simulink model "point_model"  (R2021b)
settings: Solver=VariableStepAuto  StartTime=0.0  StopTime=10.0  RelTol=1e-3
libraries: simulink_extras x4, simulink x2
settings Model: Creator=frederic  LastModifiedBy=frederic

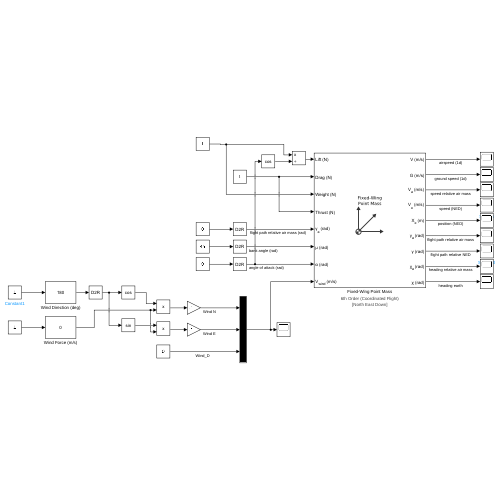
[thumbnail: Simulink's stored preview of the top-level diagram]
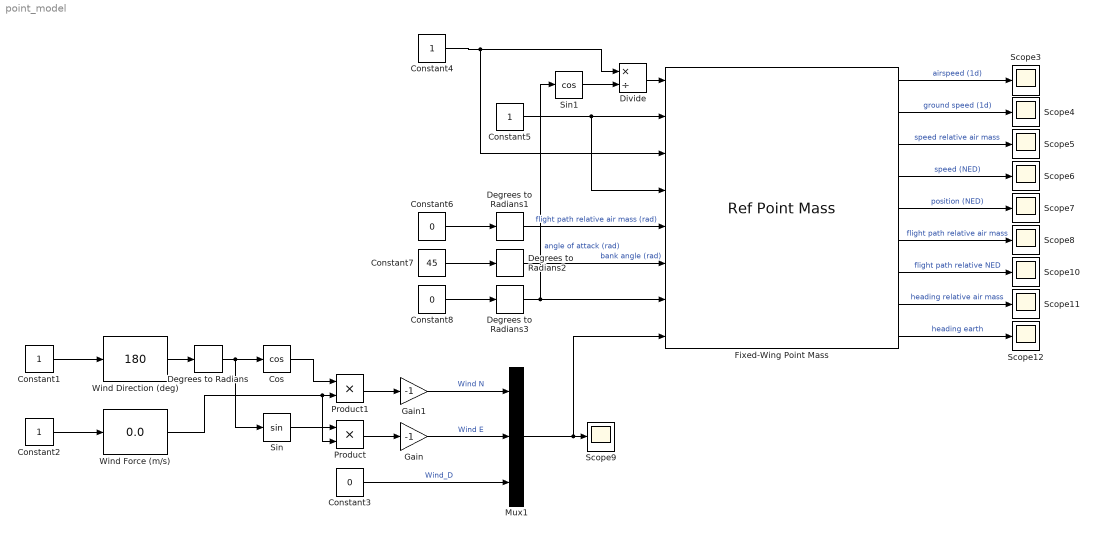
== system point_model ==
  Constant{1..2,4..5} (4 alike) : Constant
  Constant3 : Constant  Value=0
  Constant6 : Constant  Value=0
  Constant7 : Constant  Value=45
  Constant8 : Constant  Value=0
  Cos : Trigonometry  Operator=cos
  Degrees to Radians{,1..3} (4 alike) : simulink_extras/Transformations/Degrees to Radians
  Divide : Product  Inputs=*/
  Fixed-Wing Point Mass : RefPointMass  airspeed=10  mass=1
      settings: AttributesFormatString=|
      | %<order>
      | %<frame>
  Gain : Gain  Gain=-1
  Gain1 : Gain  Gain=-1
  Mux1 : Mux  Inputs=3
  Product : Product
  Product1 : Product
  Scope{3..12} (10 alike) : Scope
  Sin : Trigonometry
  Sin1 : Trigonometry  Operator=cos
  Wind Direction (deg) : simulink/Math Operations/Slider Gain  gain=180  low=0  high=359
  Wind Force (m/s) : simulink/Math Operations/Slider Gain  gain=0.0  low=0  high=30
  wires:
  Constant1/1 -> Wind Direction (deg)/1
  Constant2/1 -> Wind Force (m/s)/1
  Wind Direction (deg)/1 -> Degrees to Radians/1
  Degrees to Radians/1 -> Sin/1, Cos/1
  Sin/1 -> Product/1
  Cos/1 -> Product1/1
  Wind Force (m/s)/1 -> Product1/2, Product/2
  Product/1 -> Gain/1
  Constant3/1 -> Mux1/3  "Wind_D"
  Product1/1 -> Gain1/1
  Gain1/1 -> Mux1/1  "Wind N"
  Mux1/1 -> Fixed-Wing Point Mass/8, Scope9/1
  Gain/1 -> Mux1/2  "Wind E"
  Constant4/1 -> Fixed-Wing Point Mass/3, Divide/1
  Constant5/1 -> Fixed-Wing Point Mass/2, Fixed-Wing Point Mass/4
  Degrees to Radians1/1 -> Fixed-Wing Point Mass/5  "flight path relative air mass (rad)"
  Constant6/1 -> Degrees to Radians1/1
  Constant7/1 -> Degrees to Radians2/1
  Degrees to Radians2/1 -> Fixed-Wing Point Mass/6  "bank angle (rad)"
  Degrees to Radians3/1 -> Sin1/1, Fixed-Wing Point Mass/7  "angle of attack (rad)"
  Constant8/1 -> Degrees to Radians3/1
  Fixed-Wing Point Mass/1 -> Scope3/1  "airspeed (1d)"
  Fixed-Wing Point Mass/2 -> Scope4/1  "ground speed (1d)"
  Fixed-Wing Point Mass/3 -> Scope5/1  "speed relative air mass"
  Fixed-Wing Point Mass/4 -> Scope6/1  "speed (NED)"
  Fixed-Wing Point Mass/5 -> Scope7/1  "position (NED)"
  Fixed-Wing Point Mass/6 -> Scope8/1  "flight path relative air mass"
  Fixed-Wing Point Mass/7 -> Scope10/1  "flight path relative NED"
  Fixed-Wing Point Mass/8 -> Scope11/1  "heading relative air mass"
  Fixed-Wing Point Mass/9 -> Scope12/1  "heading earth"
  Divide/1 -> Fixed-Wing Point Mass/1
  Sin1/1 -> Divide/2
